simulink model "uav"  (Simulink 7.9)
settings: Solver=ode4  StartTime=0.0  StopTime=30  FixedStep=0.001  MinStep=0.001  RelTol=1e-3
values from neighbouring files (symbols this model uses):
  b = 10    [initialize.m]    (also in parameters.mat; uav_con.m = 8)
  d1 = 0.4    [initialize.m]    (also in parameters.mat; uav_con.m = 0.35)
  d2 = 0    [initialize.m]    (also in parameters.mat; uav_con.m)
  d3 = -0.3    [initialize.m]    (also in parameters.mat; uav_con.m = 0.3)
  jx = 0.02    [initialize.m]    (also in parameters.mat)
  jy = 0.02    [initialize.m]    (also in parameters.mat)
  jz = 0.01    [initialize.m]    (also in parameters.mat)
  k = 15    [initialize.m]    (also in parameters.mat; uav_con.m = 4)
  k_w = 0    [initialize.m]    (also in parameters.mat)
  k_w_d = 0    [initialize.m]    (also in parameters.mat)
  m = 0.5    [initialize.m]    (also in parameters.mat; uav_con.m = u(42))
  w = [inputs(7) inputs(8) inputs(9)]'    [Environment.m]    (also in initialize.m = -1; parameters.mat = -1; uav_con.m = [u(27) u(28) u(29)]'; uav_dyn.m = [x(7) x(8) x(9)]')
  w1 = 0.5    [initialize.m]    (also in parameters.mat)
  w21 = 0.3    [initialize.m]    (also in parameters.mat)
  w22 = -0.3    [initialize.m]    (also in parameters.mat)
settings Model: Creator=djlee  LastModifiedBy=user
settings SolverCC: InitialStep=0.001
settings OptimizationCC: InitFltsAndDblsToZero=on
settings DebuggingCC: SaveWithParameterizedLinksMsg=none  SignalResolutionControl=TryResolveAllWithWarning  MultiTaskDSMMsg=warning  MultiTaskCondExecSysMsg=none
settings RTWCC: IncludeERTFirstTime=on
settings CodeAppCC: CustomSymbolStrType=$N$R$M_T
settings GRTTargetCC: TargetFcnLib=ansi_tfl_tmw.mat  CombineOutputUpdateFcns=off  GRTInterface=on

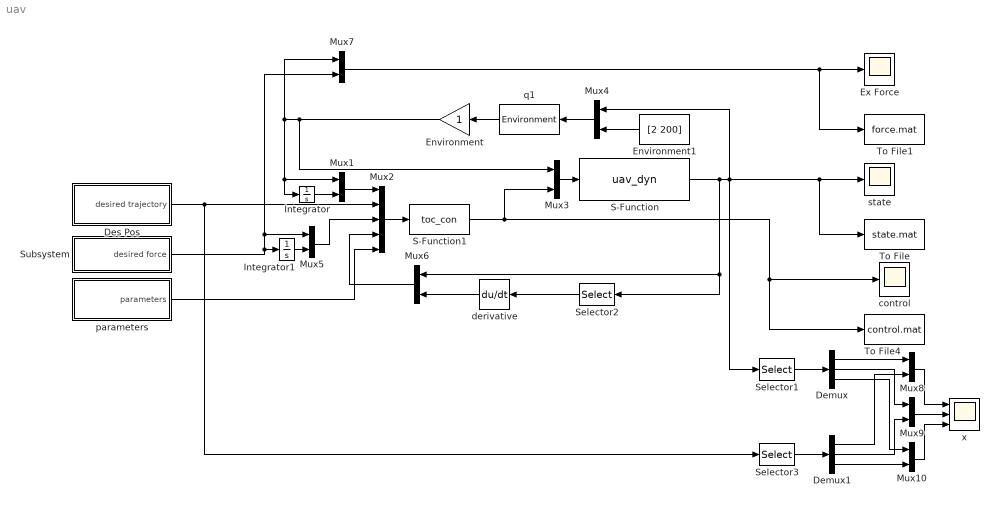
== system uav ==
  Demux : Demux  Outputs=3
  Demux1 : Demux  Outputs=3
  Des Pos : Subsystem
  Environment : Gain
  Environment1 : Constant  Value=[2 200]
  Ex Force : Scope
      settings: TimeRange=10  YMin=-2.5  YMax=0  SaveName=fe_plot
  Integrator : Integrator
  Integrator1 : Integrator
  Mux{1,3..10} (9 alike) : Mux  Inputs=2
  Mux2 : Mux  Inputs=5
  S-Function : S-Function  FunctionName=uav_dyn  Parameters=0,0,0, 1-d1,-d2,-d3, 0,0,0,0,0,0,d1,d2,d3,m,jx,jy,jz  EnableBusSupport=off
  S-Function1 : S-Function  FunctionName=toc_con  EnableBusSupport=off
  Selector1 : Selector  InputPortWidth=18  IndexOptions=Index vector (dialog)  Indices=[4:6]  OutputSizes=1
  Selector2 : Selector  InputPortWidth=18  IndexOptions=Index vector (dialog)  Indices=[1:3]  OutputSizes=1
  Selector3 : Selector  InputPortWidth=12  IndexOptions=Index vector (dialog)  Indices=[1:3]  OutputSizes=1
  Subsystem : Subsystem
  To File : ToFile  Filename=state.mat  MatrixName=state
  To File1 : ToFile  Filename=force.mat  MatrixName=force
  To File4 : ToFile  Filename=control.mat  MatrixName=control
  control : Scope
      settings: TimeRange=10  YMin=-0.5  YMax=6  SaveName=state2
  derivative : Derivative
  parameters : Subsystem
  q1 : MATLABFcn  MATLABFcn=Environment  OutputDimensions=3
  state : Scope
      settings: TimeRange=10  YMin=-7.5  YMax=7.5  SaveName=state
  x : Scope  NumInputPorts=3
      settings: TimeRange=10  YMin=1.2~-0.2~-0.8  YMax=1.2~0.8~0.2  SaveName=state1
  wires:
  Mux3/1 -> S-Function/1
  Environment/1 -> Mux3/1, Integrator/1, Mux1/1, Mux7/1
  q1/1 -> Environment/1
  Mux4/1 -> q1/1
  S-Function/1 -> Mux4/1, Mux6/1, Selector2/1, Selector1/1, state/1, To File/1
  Des Pos/1(desired trajectory) -> Mux2/2, Selector3/1
  Environment1/1 -> Mux4/2
  Integrator/1 -> Mux1/2
  Mux1/1 -> Mux2/1
  Integrator1/1 -> Mux5/2
  Mux5/1 -> Mux2/3
  Selector2/1 -> derivative/1
  derivative/1 -> Mux6/2
  Mux6/1 -> Mux2/4
  Subsystem/1(desired force) -> Integrator1/1, Mux5/1, Mux7/2
  Mux7/1 -> To File1/1, Ex Force/1
  Selector1/1 -> Demux/1
  Selector3/1 -> Demux1/1
  Demux1/1 -> Mux8/2
  Demux/1 -> Mux8/1
  Mux8/1 -> x/1
  Mux9/1 -> x/2
  Mux10/1 -> x/3
  Demux/2 -> Mux9/1
  Demux1/2 -> Mux9/2
  Demux/3 -> Mux10/1
  Demux1/3 -> Mux10/2
  parameters/1(parameters) -> Mux2/5
  Mux2/1 -> S-Function1/1
  S-Function1/1 -> Mux3/2, control/1, To File4/1

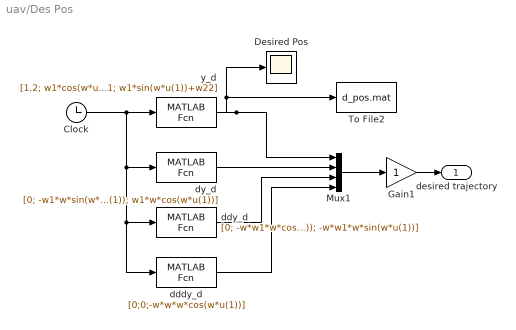
== system uav/Des Pos ==
  Clock : Clock
  Desired Pos : Scope
      settings: SaveName=y_d
  Gain1 : Gain
  Mux1 : Mux
  To File2 : ToFile  Filename=d_pos.mat  MatrixName=d_pos
  dddy_d : MATLABFcn  MATLABFcn=[0;0;-w*w*w*cos(w*u(1))]  OutputDimensions=3
  ddy_d : MATLABFcn  MATLABFcn=[0; -w*w1*w*cos(w*u(1)); -w*w1*w*sin(w*u(1))]  OutputDimensions=3
  dy_d : MATLABFcn  MATLABFcn=[0; -w1*w*sin(w*u(1)); w1*w*cos(w*u(1))]  OutputDimensions=3
  y_d : MATLABFcn  MATLABFcn=[1.2; w1*cos(w*u(1))+w21; w1*sin(w*u(1))+w22]  OutputDimensions=3  Output1D=off
  desired trajectory : Outport
  wires:
  dy_d/1 -> Mux1/2
  ddy_d/1 -> Mux1/3
  Mux1/1 -> Gain1/1
  y_d/1 -> Mux1/1, Desired Pos/1, To File2/1
  Clock/1 -> dy_d/1, ddy_d/1, dddy_d/1, y_d/1
  Gain1/1 -> desired trajectory/1
  dddy_d/1 -> Mux1/4

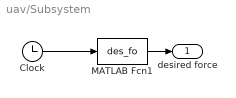
== system uav/Subsystem ==
  Clock : Clock
  MATLAB Fcn1 : MATLABFcn  MATLABFcn=des_fo  OutputDimensions=1  Output1D=off
  desired force : Outport
  wires:
  Clock/1 -> MATLAB Fcn1/1
  MATLAB Fcn1/1 -> desired force/1

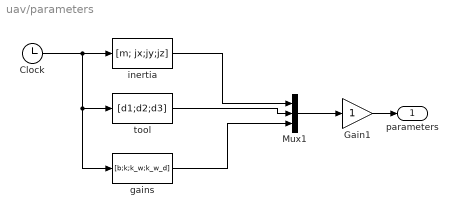
== system uav/parameters ==
  Clock : Clock
  Gain1 : Gain
  Mux1 : Mux  Inputs=3
  gains : MATLABFcn  MATLABFcn=[b;k;k_w;k_w_d]  OutputDimensions=4
  inertia : MATLABFcn  MATLABFcn=[m; jx;jy;jz]  OutputDimensions=4  Output1D=off
  tool : MATLABFcn  MATLABFcn=[d1;d2;d3]  OutputDimensions=3
  parameters : Outport
  wires:
  tool/1 -> Mux1/2
  Mux1/1 -> Gain1/1
  inertia/1 -> Mux1/1
  Clock/1 -> inertia/1, tool/1, gains/1
  Gain1/1 -> parameters/1
  gains/1 -> Mux1/3
